simulink model "product"  (Simulink 7.3)
settings: Solver=FixedStepDiscrete  StartTime=0.0  StopTime=10.0  FixedStep=1  RelTol=1e-3
settings Model: Creator=Nyenyec  LastModifiedBy=hnine
settings OptimizationCC: InitFltsAndDblsToZero=on
settings DebuggingCC: SaveWithParameterizedLinksMsg=none
settings GRTTargetCC: TargetFcnLib=ansi_tfl_tmw.mat

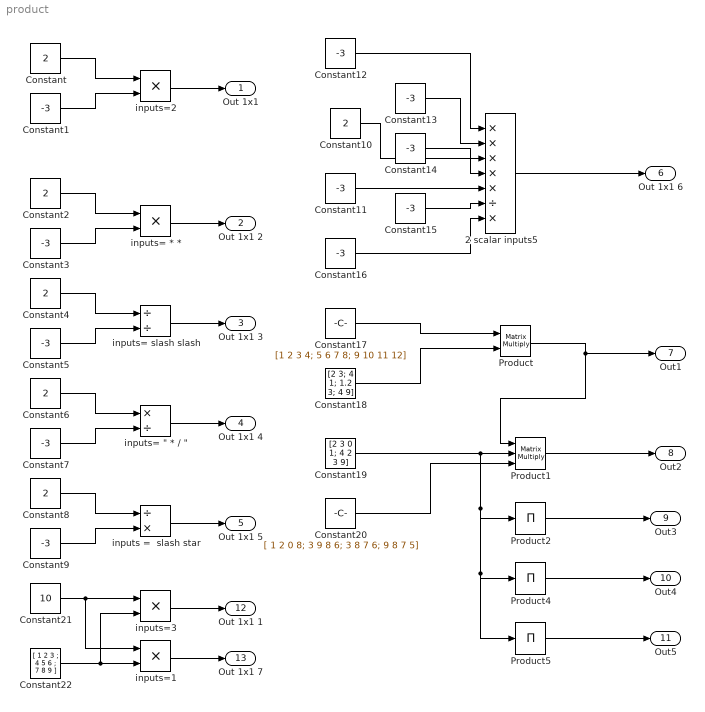
== system product ==
  2 scalar inputs5 : Product  Inputs=*****/*  OutDataType=sfix(16)  OutScaling=2^0  RndMeth=Zero
  Constant{,2,4,6,8,10} (6 alike) : Constant  Value=2  OutDataType=sfix(16)  OutScaling=2^0
  Constant{1,3,5,7,9,11..16} (11 alike) : Constant  Value=-3  OutDataType=sfix(16)  OutScaling=2^0
  Constant17 : Constant  Value=[1 2 3 4; 5 6 7 8; 9 10 11 12]  OutDataType=sfix(16)  OutScaling=2^0
  Constant18 : Constant  Value=[2 3; 4 1; 1.2 3; 4 9]  OutDataType=sfix(16)  OutScaling=2^0
  Constant19 : Constant  Value=[2 3 0 1; 4 2 3 9]  OutDataType=sfix(16)  OutScaling=2^0
  Constant20 : Constant  Value=[ 1 2 0 8; 3 9 8 6; 3 8 7 6; 9 8 7 5]  OutDataType=sfix(16)  OutScaling=2^0
  Constant21 : Constant  Value=10  OutDataType=sfix(16)  OutScaling=2^0
  Constant22 : Constant  Value=[ 1 2 3 ; 4 5 6 ; 7 8 9 ]  OutDataType=sfix(16)  OutScaling=2^0
  Product : Product  Multiplication=Matrix(*)  OutDataType=sfix(16)  OutScaling=2^0  RndMeth=Zero
  Product1 : Product  Inputs=3  Multiplication=Matrix(*)  OutDataType=sfix(16)  OutScaling=2^0  RndMeth=Zero
  Product2 : Product  Inputs=1  OutDataType=sfix(16)  OutScaling=2^0  RndMeth=Zero
  Product4 : Product  Inputs=1  CollapseMode=Specified dimension  OutDataType=sfix(16)  OutScaling=2^0  RndMeth=Zero
  Product5 : Product  Inputs=1  CollapseMode=Specified dimension  CollapseDim=2  OutDataType=sfix(16)  OutScaling=2^0  RndMeth=Zero
  inputs =  slash star : Product  Inputs=/*  OutDataType=sfix(16)  OutScaling=2^0  RndMeth=Zero
  "inputs= \" * / \"" : Product  Inputs=*/  OutDataType=sfix(16)  OutScaling=2^0  RndMeth=Zero
  inputs= * * : Product  Inputs=**  OutDataType=sfix(16)  OutScaling=2^0  RndMeth=Zero
  inputs= slash slash : Product  Inputs=//  OutDataType=sfix(16)  OutScaling=2^0  RndMeth=Zero
  inputs=1 : Product  OutDataType=sfix(16)  OutScaling=2^0  RndMeth=Zero
  inputs=2 : Product  OutDataType=sfix(16)  OutScaling=2^0  RndMeth=Zero
  inputs=3 : Product  OutDataType=sfix(16)  OutScaling=2^0  RndMeth=Zero
  Out 1x1 : Outport  OutDataType=sfix(16)  OutScaling=2^0
  Out 1x1 2 : Outport  Port=2  OutDataType=sfix(16)  OutScaling=2^0
  Out 1x1 3 : Outport  Port=3  OutDataType=sfix(16)  OutScaling=2^0
  Out 1x1 4 : Outport  Port=4  OutDataType=sfix(16)  OutScaling=2^0
  Out 1x1 5 : Outport  Port=5  OutDataType=sfix(16)  OutScaling=2^0
  Out 1x1 6 : Outport  Port=6  OutDataType=sfix(16)  OutScaling=2^0
  Out1 : Outport  Port=7  OutDataType=sfix(16)  OutScaling=2^0
  Out2 : Outport  Port=8  OutDataType=sfix(16)  OutScaling=2^0
  Out3 : Outport  Port=9  OutDataType=sfix(16)  OutScaling=2^0
  Out4 : Outport  Port=10  OutDataType=sfix(16)  OutScaling=2^0
  Out5 : Outport  Port=11  OutDataType=sfix(16)  OutScaling=2^0
  Out 1x1 1 : Outport  Port=12  OutDataType=sfix(16)  OutScaling=2^0
  Out 1x1 7 : Outport  Port=13  OutDataType=sfix(16)  OutScaling=2^0
  wires:
  Constant/1 -> inputs=2/1
  Constant1/1 -> inputs=2/2
  inputs=2/1 -> Out 1x1/1
  Constant2/1 -> inputs= * */1
  Constant3/1 -> inputs= * */2
  inputs= * */1 -> Out 1x1 2/1
  Constant4/1 -> inputs= slash slash/1
  Constant5/1 -> inputs= slash slash/2
  inputs= slash slash/1 -> Out 1x1 3/1
  Constant6/1 -> "inputs= \" * / \""/1
  Constant7/1 -> "inputs= \" * / \""/2
  "inputs= \" * / \""/1 -> Out 1x1 4/1
  Constant8/1 -> inputs =  slash star/1
  Constant9/1 -> inputs =  slash star/2
  inputs =  slash star/1 -> Out 1x1 5/1
  Constant12/1 -> 2 scalar inputs5/1
  Constant13/1 -> 2 scalar inputs5/2
  Constant10/1 -> 2 scalar inputs5/3
  Constant14/1 -> 2 scalar inputs5/4
  Constant11/1 -> 2 scalar inputs5/5
  Constant15/1 -> 2 scalar inputs5/6
  Constant16/1 -> 2 scalar inputs5/7
  2 scalar inputs5/1 -> Out 1x1 6/1
  Constant17/1 -> Product/1
  Product/1 -> Out1/1, Product1/1
  Constant18/1 -> Product/2
  Constant19/1 -> Product1/2, Product2/1, Product4/1, Product5/1
  Product1/1 -> Out2/1
  Constant20/1 -> Product1/3
  Product2/1 -> Out3/1
  Product4/1 -> Out4/1
  Product5/1 -> Out5/1
  Constant21/1 -> inputs=3/1, inputs=1/1
  Constant22/1 -> inputs=1/2, inputs=3/2
  inputs=3/1 -> Out 1x1 1/1
  inputs=1/1 -> Out 1x1 7/1
